simulink model "Lab4"  (R2018a)
settings: Solver=VariableStepAuto  StartTime=0.0  StopTime=10.0  RelTol=1e-3
values from neighbouring files (symbols this model uses):
  A = [(2*s+3+(10/s)) -((5/(s))+3);      -(3+(5/(s))) (2*s + 6 +(5/s))]    [Lab2.m]    (also in Lab_4.m = [0  1 0 0; ((M+m)*g)/(M*L) 0 0 0;     0 0 0 1; -m*g/M 0 0 0]; l77.m = [0 1 0; 0 0 1; -501.6*10^-6 -128.8*10^-3  -854*10^-3])
  B = [10;0]    [Lab2.m]    (also in Lab_4.m = [0;-1/(M*L); 0; 1/M]; l77.m = [1 0 0]')
  C = [L 0 1 0]    [Lab_4.m]    (also in l77.m = [0.78*10^-4 4.14*10^-4 0.01])
  D = 0    [Lab_4.m]    (also in l77.m)
settings Model: Creator=sephella  LastModifiedBy=sephella

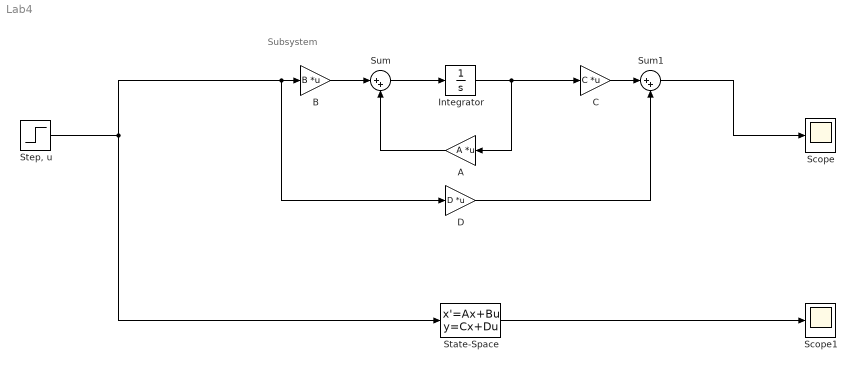
== system Lab4 ==
  note: Subsystem
  A : Gain  Gain=A  Multiplication=Matrix(K*u)
  B : Gain  Gain=B  Multiplication=Matrix(K*u)
  C : Gain  Gain=C  Multiplication=Matrix(K*u)
  D : Gain  Gain=D  Multiplication=Matrix(K*u)
  Integrator : Integrator
  Scope : Scope
  Scope1 : Scope
  State-Space : StateSpace  A=A  B=B  C=C  D=D  InitialCondition=0
  "Step, u " : Step  Time=0  SampleTime=0
  Sum : Sum  Inputs=|++
  Sum1 : Sum  Inputs=|++
  wires:
  Sum1/1 -> Scope/1
  State-Space/1 -> Scope1/1
  C/1 -> Sum1/1
  Integrator/1 -> A/1, C/1
  D/1 -> Sum1/2
  A/1 -> Sum/2
  "Step, u "/1 -> D/1, B/1, State-Space/1
  B/1 -> Sum/1
  Sum/1 -> Integrator/1
